simulink model "MPC_fmin_implemented"  (R2016b)
settings: Solver=VariableStepAuto  StartTime=0.0  StopTime=100  RelTol=1e-3
values from neighbouring files (symbols this model uses):
  a = 5.713e-09    [LQI_script.m]    (also in PID_script.m = 4.367e-09; fminsim.m = block.InputPort(3).Data; model_generation.m = 4.367e-09)
  b = 0.000324    [LQI_script.m]    (also in PID_script.m = 0.0002827; fminsim.m = block.InputPort(4).Data; model_generation.m = 0.0002827)
  m = 56.3/1000    (= 0.0563)    [LQI_script.m]    (also in PID_script.m; model_generation.m)
  x0 = 0.002    [model_generation.m]    (also in sfserialout.m = [])
  x1 = 0.02525    [LQI_script.m]    (also in PID_script.m; fminsim.m = block.InputPort(5).Data; model_generation.m)
  x2 = 0.05    [LQI_script.m]    (also in PID_script.m; fminsim.m = block.InputPort(6).Data; model_generation.m)
  x3 = 0.0751    [LQI_script.m]    (also in PID_script.m; fminsim.m = block.InputPort(7).Data; model_generation.m)
  x4 = 0.103    [LQI_script.m]    (also in PID_script.m; fminsim.m = block.InputPort(8).Data; model_generation.m)
libraries: mpclib x1
settings Model: Creator=fly_a  LastModifiedBy=fly_a

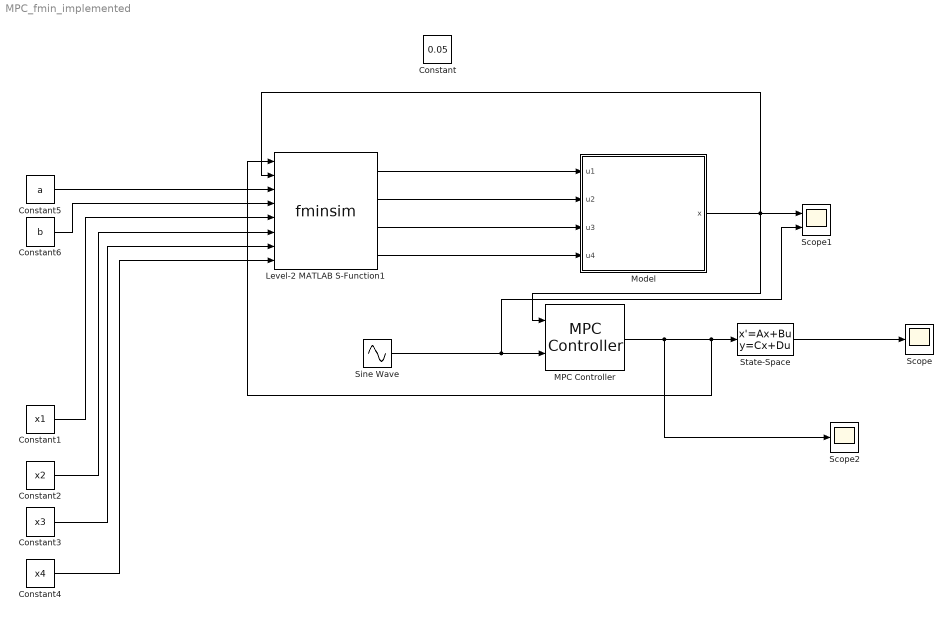
== system MPC_fmin_implemented ==
  Constant : Constant  Value=0.05
  Constant1 : Constant  Value=x1
  Constant2 : Constant  Value=x2
  Constant3 : Constant  Value=x3
  Constant4 : Constant  Value=x4
  Constant5 : Constant  Value=a
  Constant6 : Constant  Value=b
  Level-2 MATLAB S-Function1 : M-S-Function  FunctionName=fminsim
  MPC Controller : mpclib/MPC Controller  SCDEnableBlockLinearizationSpecification=on  mpcobj=mpc1  is_multiple=0  enable_value=0  return_u0=off  ref_from_ws=off  ref_signal_name=[]  ref_preview=off  md_from_ws=off  md_signal_name=[]  md_preview=off  from_project=off  project_file=MPCtask.mat  md_inport=off  mv_inport=off  cost_outport=off  return_sequence=off  return_qpstatus=off  return_state=off  state_inport=off  lims_inport=off  ywt_inport=off  is_designfromscratch=0  uwt_inport=off  duwt_inport=off  rhoeps_inport=off  uref_inport=off  n_ts=0.1  n_mv=1  n_md=0  n_ud=0  n_mo=1  n_uo=0  BlockDataType=double  SampleTimeInherited=off  switch_inport=off
  Model : Subsystem
  Scope : Scope
  Scope1 : Scope  NumInputPorts=2
  Scope2 : Scope
  Sine Wave : Sin  Amplitude=0.02  Bias=0.04  Frequency=0.01  SampleTime=0
  State-Space : StateSpace  A=[ 0 1; 0 0 ]  B=[ 0 ; 1/m]  C=[ 1 0 ]  D=[0]  X0=[ 0; 0]
  wires:
  State-Space/1 -> Scope/1
  Sine Wave/1 -> Scope1/2, MPC Controller/2
  Constant4/1 -> Level-2 MATLAB S-Function1/8
  Constant3/1 -> Level-2 MATLAB S-Function1/7
  Constant2/1 -> Level-2 MATLAB S-Function1/6
  Constant1/1 -> Level-2 MATLAB S-Function1/5
  Constant6/1 -> Level-2 MATLAB S-Function1/4
  Constant5/1 -> Level-2 MATLAB S-Function1/3
  MPC Controller/1 -> Scope2/1, Level-2 MATLAB S-Function1/1, State-Space/1
  Level-2 MATLAB S-Function1/1 -> Model/1(u1)
  Level-2 MATLAB S-Function1/2 -> Model/2(u2)
  Level-2 MATLAB S-Function1/3 -> Model/3(u3)
  Level-2 MATLAB S-Function1/4 -> Model/4(u4)
  Model/1(x) -> MPC Controller/1, Scope1/1, Level-2 MATLAB S-Function1/2

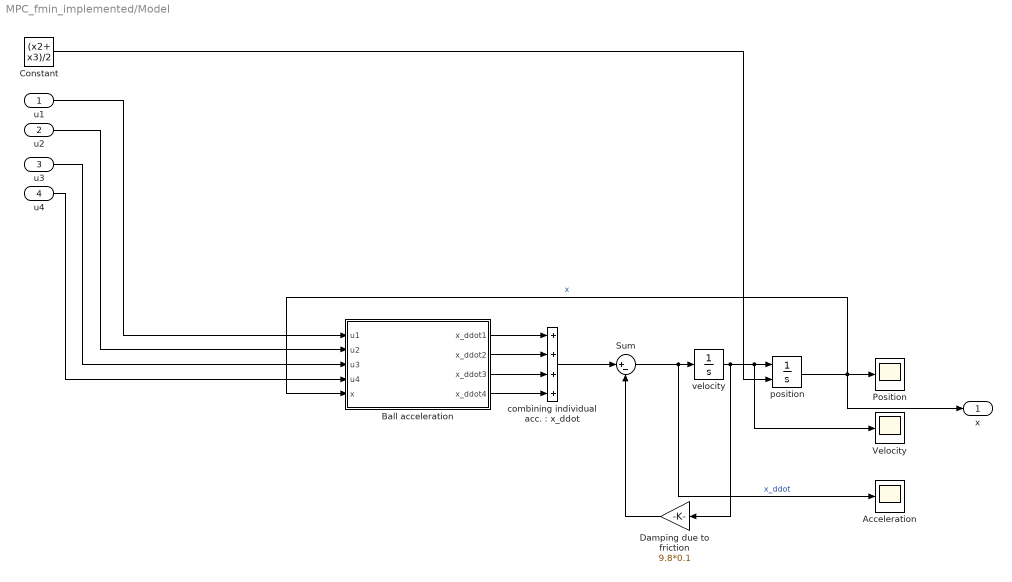
== system MPC_fmin_implemented/Model ==
  u1 : Inport
  u2 : Inport  Port=2
  u3 : Inport  Port=3
  u4 : Inport  Port=4
  Acceleration : Scope
  Ball acceleration : Subsystem
  Constant : Constant  Value=(x2+ x3)/2
  Damping due to friction : Gain  Gain=9.8*0.1
  Position : Scope
  Sum : Sum  Inputs=|+-
  Velocity : Scope
  "combining individual acc. : x_ddot" : Sum  Inputs=++++
  position : Integrator  InitialConditionSource=external  InitialCondition=x0
  velocity : Integrator
  x : Outport
  wires:
  Ball acceleration/1(x_ddot1) -> "combining individual acc. : x_ddot"/1
  Ball acceleration/2(x_ddot2) -> "combining individual acc. : x_ddot"/2
  Ball acceleration/3(x_ddot3) -> "combining individual acc. : x_ddot"/3
  Ball acceleration/4(x_ddot4) -> "combining individual acc. : x_ddot"/4
  velocity/1 -> Velocity/1, position/1, Damping due to friction/1
  position/1 -> Ball acceleration/5(x), Position/1, x/1  "x"
  "combining individual acc. : x_ddot"/1 -> Sum/1
  Sum/1 -> Acceleration/1, velocity/1  "x_ddot"
  Damping due to friction/1 -> Sum/2
  u1/1 -> Ball acceleration/1(u1)
  u2/1 -> Ball acceleration/2(u2)
  u3/1 -> Ball acceleration/3(u3)
  u4/1 -> Ball acceleration/4(u4)
  Constant/1 -> position/2

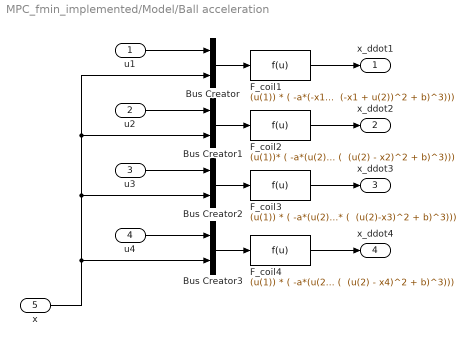
== system MPC_fmin_implemented/Model/Ball acceleration ==
  u1 : Inport
  u2 : Inport  Port=2
  u3 : Inport  Port=3
  u4 : Inport  Port=4
  x : Inport  Port=5
  Bus Creator{,1..3} (4 alike) : BusCreator  Inputs=2
  F_coil1 : Fcn  Expr="(u(1)) * ( -a*(-x1+u(2)) / ( (m* (  (-x1 + u(2))^2 + b)^3)))"
  F_coil2 : Fcn  Expr="(u(1))* ( -a*(u(2)-x2) / ( (m* (  (u(2) - x2)^2 + b)^3)))"
  F_coil3 : Fcn  Expr="(u(1)) * ( -a*(u(2)-x3) / ( (m* (  (u(2)-x3)^2 + b)^3)))"
  F_coil4 : Fcn  Expr="(u(1)) * ( -a*(u(2) -x4 ) / ( (m* (  (u(2) - x4)^2 + b)^3)))"
  x_ddot1 : Outport
  x_ddot2 : Outport  Port=2
  x_ddot3 : Outport  Port=3
  x_ddot4 : Outport  Port=4
  wires:
  F_coil1/1 -> x_ddot1/1
  F_coil2/1 -> x_ddot2/1
  F_coil3/1 -> x_ddot3/1
  F_coil4/1 -> x_ddot4/1
  x/1 -> Bus Creator/2, Bus Creator1/2, Bus Creator2/2, Bus Creator3/2
  Bus Creator/1 -> F_coil1/1
  u1/1 -> Bus Creator/1
  Bus Creator1/1 -> F_coil2/1
  u2/1 -> Bus Creator1/1
  u3/1 -> Bus Creator2/1
  Bus Creator2/1 -> F_coil3/1
  u4/1 -> Bus Creator3/1
  Bus Creator3/1 -> F_coil4/1
